simulink subsystem "ConfiguredSimulinkPlantModels"  (R2023a)
settings: Solver=VariableStepAuto  StartTime=0.0  StopTime=10.0  RelTol=1e-3
undefined symbols (not defined in the file or in its folder): PlntDCDCVoltInit, PlntTrnsfrCaseAxlSpdLock, PlntTrnsfrCaseTrqSplitRatio
(part 2 of 2)

== system ConfiguredSimulinkPlantModels/Electrical System/Electrical System/Battery System ==
  note: 1) Add Subsystem or Model blocks as valid variant choices.
      | 2) You cannot connect blocks at this level. At simulation, connectivity is automatically
      | determined, based on the active variant and port name matching.
  LdCurr : Inport
  BattTemp : Inport  Port=2
  Mapped Battery : Subsystem  VariantControl=Mapped Battery  ReferencedSubsystem=Battery
  BattSoc : Outport  VectorParamsAs1DForOutWhenUnconnected=off
  BattCurr : Outport  Port=2  VectorParamsAs1DForOutWhenUnconnected=off
  BattVolt : Outport  Port=3  VectorParamsAs1DForOutWhenUnconnected=off
  BMSSensors : Outport  Port=4  VectorParamsAs1DForOutWhenUnconnected=off

== system ConfiguredSimulinkPlantModels/Electrical System/Electrical System/DC-DC Converter ==
  BatVolt : Inport
  LdCurr : Inport  Port=2
  VoltCmd : Inport  Port=3
  DC-DC Converter : Subsystem  VariantControl=DC-DC Converter  ReferencedSubsystem=DCDCConverter
  No DC-DC Converter : Subsystem  VariantControl=No DC-DC Converter  ReferencedSubsystem=NoDCDCConverter
  BusVolt : Outport
  SrcCurr : Outport  Port=2

== system ConfiguredSimulinkPlantModels/Electrical System/Electrical System/Electric Machines ==
  EMTrqCmd : Inport
  EMSpd : Inport  Port=2
  BusVolt : Inport  Port=3
  2EM : Subsystem  VariantControl=2EM
  EMTrq : Outport
  EMPwrElec : Outport  Port=2
  EMCurr : Outport  Port=3

== system ConfiguredSimulinkPlantModels/Electrical System/Electrical System 1EM/Battery System ==
  note: 1) Add Subsystem or Model blocks as valid variant choices.
      | 2) You cannot connect blocks at this level. At simulation, connectivity is automatically
      | determined, based on the active variant and port name matching.
  LdCurr : Inport
  BattTemp : Inport  Port=2
  Ideal Voltage Source : Subsystem  VariantControl=Ideal Voltage Source  ReferencedSubsystem=IdealVoltageSource
  Mapped Battery : Subsystem  VariantControl=Mapped Battery  ReferencedSubsystem=Battery
  BattSoc : Outport  VectorParamsAs1DForOutWhenUnconnected=off
  BattCurr : Outport  Port=2  VectorParamsAs1DForOutWhenUnconnected=off
  BattVolt : Outport  Port=3  VectorParamsAs1DForOutWhenUnconnected=off
  BMSSensors : Outport  Port=4  VectorParamsAs1DForOutWhenUnconnected=off

== system ConfiguredSimulinkPlantModels/Electrical System/Electrical System 1EM/DC-DC Converter ==
  BatVolt : Inport
  LdCurr : Inport  Port=2
  VoltCmd : Inport  Port=3
  DC-DC Converter : Subsystem  VariantControl=DC-DC Converter  ReferencedSubsystem=DCDCConverter
  No DC-DC Converter : Subsystem  VariantControl=No DC-DC Converter  ReferencedSubsystem=NoDCDCConverter
  BusVolt : Outport
  SrcCurr : Outport  Port=2

== system ConfiguredSimulinkPlantModels/Electrical System/Electrical System 1EM/Electric Machine 1 ==
  EMTrqCmd : Inport
  EMSpd : Inport  Port=2
  BusVolt : Inport  Port=3
  Mapped EM : Subsystem  VariantControl=Mapped EM  ReferencedSubsystem=ElectricMachine1
  EMTrq : Outport  VectorParamsAs1DForOutWhenUnconnected=off
  EMCurr : Outport  Port=2  VectorParamsAs1DForOutWhenUnconnected=off

== system ConfiguredSimulinkPlantModels/Electrical System/Electrical System 2EM/Battery System ==
  note: 1) Add Subsystem or Model blocks as valid variant choices.
      | 2) You cannot connect blocks at this level. At simulation, connectivity is automatically
      | determined, based on the active variant and port name matching.
  LdCurr : Inport
  BattTemp : Inport  Port=2
  Ideal Voltage Source : Subsystem  VariantControl=Ideal Voltage Source  ReferencedSubsystem=IdealVoltageSource
  Mapped Battery : Subsystem  VariantControl=Mapped Battery  ReferencedSubsystem=Battery
  BattSoc : Outport  VectorParamsAs1DForOutWhenUnconnected=off
  BattCurr : Outport  Port=2  VectorParamsAs1DForOutWhenUnconnected=off
  BattVolt : Outport  Port=3  VectorParamsAs1DForOutWhenUnconnected=off
  BMSSensors : Outport  Port=4  VectorParamsAs1DForOutWhenUnconnected=off

== system ConfiguredSimulinkPlantModels/Electrical System/Electrical System 2EM/DC-DC Converter ==
  BatVolt : Inport
  LdCurr : Inport  Port=2
  VoltCmd : Inport  Port=3
  DC-DC Converter : Subsystem  VariantControl=DC-DC Converter  ReferencedSubsystem=DCDCConverter
  No DC-DC Converter : Subsystem  VariantControl=No DC-DC Converter  ReferencedSubsystem=NoDCDCConverter
  BusVolt : Outport
  SrcCurr : Outport  Port=2

== system ConfiguredSimulinkPlantModels/Electrical System/Electrical System 2EM/Electric Machine 1 ==
  EMTrqCmd : Inport
  EMSpd : Inport  Port=2
  BusVolt : Inport  Port=3
  Mapped EM : Subsystem  VariantControl=Mapped EM  ReferencedSubsystem=ElectricMachine1
  EMTrq : Outport  VectorParamsAs1DForOutWhenUnconnected=off
  EMCurr : Outport  Port=2  VectorParamsAs1DForOutWhenUnconnected=off

== system ConfiguredSimulinkPlantModels/Electrical System/Electrical System 2EM/Electric Machine 2 ==
  EMTrqCmd : Inport
  EMSpd : Inport  Port=2
  BusVolt : Inport  Port=3
  Mapped EM : Subsystem  VariantControl=Mapped EM  ReferencedSubsystem=ElectricMachine2
  EMTrq : Outport  VectorParamsAs1DForOutWhenUnconnected=off
  EMCurr : Outport  Port=2  VectorParamsAs1DForOutWhenUnconnected=off

== system ConfiguredSimulinkPlantModels/Sensors/Sensors/No IMU Sensor ==
  VehFdbk : Inport
  Bus Creator1 : BusCreator  Inputs=2
  Constant : Constant  Value=zeros(3,1)  SampleTime=-1
  Constant1 : Constant  Value=zeros(3,1)  SampleTime=-1
  Terminator : Terminator
  IMU : Outport
  wires:
  VehFdbk/1 -> Terminator/1
  Constant1/1 -> Bus Creator1/2  "pqr"
  Bus Creator1/1 -> IMU/1  "IMU"
  Constant/1 -> Bus Creator1/1  "Acc"

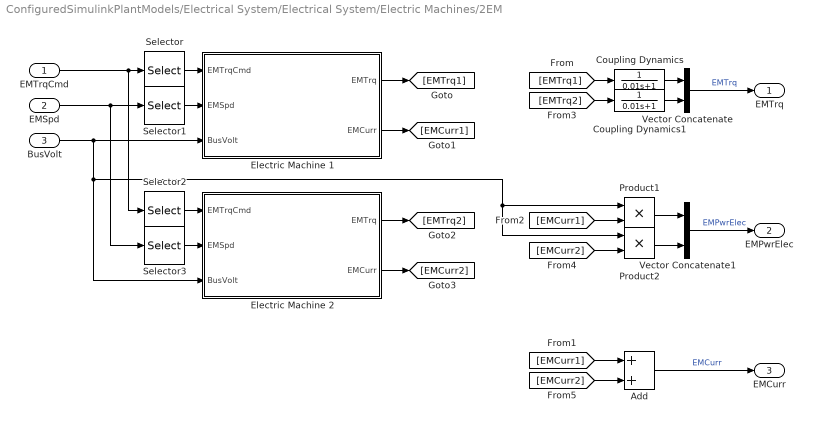
== system ConfiguredSimulinkPlantModels/Electrical System/Electrical System/Electric Machines/2EM ==
  EMTrqCmd : Inport
  EMSpd : Inport  Port=2
  BusVolt : Inport  Port=3
  Add : Sum
  Coupling Dynamics : TransferFcn  Denominator=[0.01 1]
  Coupling Dynamics1 : TransferFcn  Denominator=[0.01 1]
  Electric Machine 1 : Subsystem  Variant=on  VariantControlMode=label  LabelModeActiveChoice=Mapped EM
  Electric Machine 2 : Subsystem  Variant=on  VariantControlMode=label  LabelModeActiveChoice=Mapped EM
  Product1 : Product
  Product2 : Product
  Selector : Selector  InputPortWidth=2  IndexOptions=Index vector (dialog)  Indices=[1]  OutputSizes=1
  Selector1 : Selector  InputPortWidth=2  IndexOptions=Index vector (dialog)  Indices=[1]  OutputSizes=1
  Selector2 : Selector  InputPortWidth=2  IndexOptions=Index vector (dialog)  Indices=[2]  OutputSizes=1
  Selector3 : Selector  InputPortWidth=2  IndexOptions=Index vector (dialog)  Indices=[2]  OutputSizes=1
  Vector Concatenate : Concatenate
  Vector Concatenate1 : Concatenate
  EMTrq : Outport
  EMPwrElec : Outport  Port=2
  EMCurr : Outport  Port=3
  wires:
  Electric Machine 2/2(EMCurr) -> [EMCurr2]
  Electric Machine 2/1(EMTrq) -> [EMTrq2]
  [EMCurr2] -> Add/2
  [EMCurr2] -> Product2/2
  [EMTrq2] -> Coupling Dynamics1/1
  [EMCurr1] -> Product1/2
  [EMCurr1] -> Add/1
  Electric Machine 1/2(EMCurr) -> [EMCurr1]
  [EMTrq1] -> Coupling Dynamics/1
  Electric Machine 1/1(EMTrq) -> [EMTrq1]
  EMSpd/1 -> Selector3/1, Selector1/1
  Selector/1 -> Electric Machine 1/1(EMTrqCmd)
  Add/1 -> EMCurr/1  "EMCurr"
  Selector2/1 -> Electric Machine 2/1(EMTrqCmd)
  Coupling Dynamics1/1 -> Vector Concatenate/2
  Product2/1 -> Vector Concatenate1/2
  Product1/1 -> Vector Concatenate1/1
  EMTrqCmd/1 -> Selector2/1, Selector/1
  Selector3/1 -> Electric Machine 2/2(EMSpd)
  Selector1/1 -> Electric Machine 1/2(EMSpd)
  Vector Concatenate1/1 -> EMPwrElec/1  "EMPwrElec"
  Coupling Dynamics/1 -> Vector Concatenate/1
  BusVolt/1 -> Electric Machine 1/3(BusVolt), Electric Machine 2/3(BusVolt), Product1/1, Product2/1
  Vector Concatenate/1 -> EMTrq/1  "EMTrq"

== system ConfiguredSimulinkPlantModels/Electrical System/Electrical System/Electric Machines/2EM/Electric Machine 1 ==
  EMTrqCmd : Inport
  EMSpd : Inport  Port=2
  BusVolt : Inport  Port=3
  Mapped EM : Subsystem  VariantControl=Mapped EM  ReferencedSubsystem=ElectricMachine1
  EMTrq : Outport  VectorParamsAs1DForOutWhenUnconnected=off
  EMCurr : Outport  Port=2  VectorParamsAs1DForOutWhenUnconnected=off

== system ConfiguredSimulinkPlantModels/Electrical System/Electrical System/Electric Machines/2EM/Electric Machine 2 ==
  EMTrqCmd : Inport
  EMSpd : Inport  Port=2
  BusVolt : Inport  Port=3
  Mapped EM : Subsystem  VariantControl=Mapped EM  ReferencedSubsystem=ElectricMachine2
  EMTrq : Outport  VectorParamsAs1DForOutWhenUnconnected=off
  EMCurr : Outport  Port=2  VectorParamsAs1DForOutWhenUnconnected=off
